simulink model "simlink13"  (R2017b)
settings: Solver=VariableStepAuto  StartTime=0.0  StopTime=10  RelTol=1e-3
PreLoadFcn:
  | init.m;
settings Model: Creator=Administrator  LastModifiedBy=Administrator
settings SolverCC: ZeroCrossAlgorithm=Adaptive
settings DebuggingCC: MaxConsecutiveZCsMsg=none

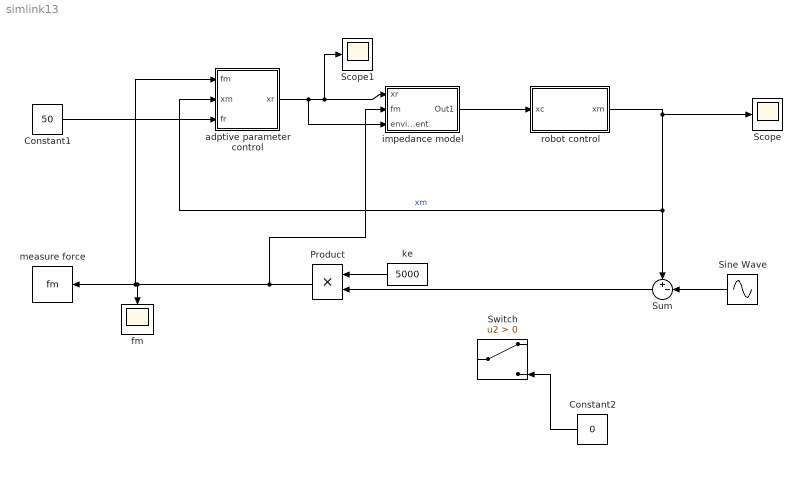
== system simlink13 ==
  Constant1 : Constant  Value=50
  Constant2 : Constant  Value=0
  Product : Product
  Scope : Scope
  Scope1 : Scope
  Sine Wave : Sin  SampleTime=0
  Sum : Sum  Inputs=+-|
  Switch : Switch  Criteria=u2 > Threshold
  adptive parameter control : Subsystem
  fm : Scope
  impedance model : Subsystem
  ke : Constant  Value=5000
  "measure force " : ToWorkspace  VariableName=fm  SaveFormat=Timeseries  SampleTime=-1
  robot control : Subsystem
  wires:
  Constant1/1 -> adptive parameter control/3(fr)
  Product/1 -> impedance model/2(fm), "measure force "/1, adptive parameter control/1(fm), fm/1
  robot control/1("xm ") -> adptive parameter control/2(xm), Sum/1, Scope/1  "xm"
  impedance model/1(Out1) -> robot control/1(xc)
  ke/1 -> Product/1
  adptive parameter control/1(xr) -> impedance model/3(envirment), Scope1/1, impedance model/1(xr)
  Sine Wave/1 -> Sum/2
  Constant2/1 -> Switch/3
  Sum/1 -> Product/2

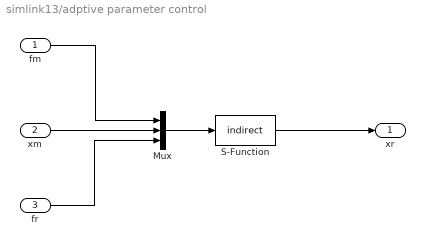
== system simlink13/adptive parameter control ==
  fm : Inport
  xm : Inport  Port=2
  fr : Inport  Port=3
  Mux : Mux  Inputs=3
  S-Function : S-Function  FunctionName=indirect  Parameters=gama1 gama2 kd  SFunctionDeploymentMode=off  EnableBusSupport=off
  xr : Outport
  wires:
  fm/1 -> Mux/1
  xm/1 -> Mux/2
  Mux/1 -> S-Function/1
  S-Function/1 -> xr/1
  fr/1 -> Mux/3

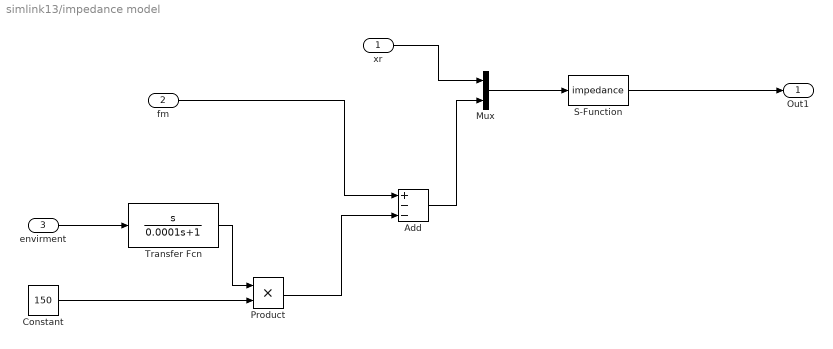
== system simlink13/impedance model ==
  xr : Inport
  fm : Inport  Port=2
  envirment : Inport  Port=3
  Add : Sum  Inputs=+--
  Constant : Constant  Value=150
  Mux : Mux  Inputs=2
  Product : Product
  S-Function : S-Function  FunctionName=impedance  Parameters=bd kd  SFunctionDeploymentMode=off  EnableBusSupport=off
  Transfer Fcn : TransferFcn  Numerator=[1 0]  Denominator=[0.0001 1]
  Out1 : Outport
  wires:
  xr/1 -> Mux/1
  Mux/1 -> S-Function/1
  S-Function/1 -> Out1/1
  Transfer Fcn/1 -> Product/1
  envirment/1 -> Transfer Fcn/1
  Add/1 -> Mux/2
  Constant/1 -> Product/2
  fm/1 -> Add/1
  Product/1 -> Add/3

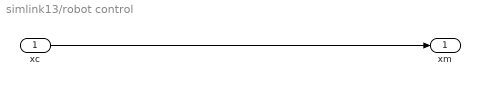
== system simlink13/robot control ==
  xc : Inport
  "xm " : Outport
  wires:
  xc/1 -> "xm "/1
